simulink model "population_fractal"  (Simulink 7.1)
settings: Solver=ode45  StartTime=0.0  StopTime=600.0  RelTol=1e-3
libraries: simulink x1
settings Model: Creator=Usuario  LastModifiedBy=Usuario

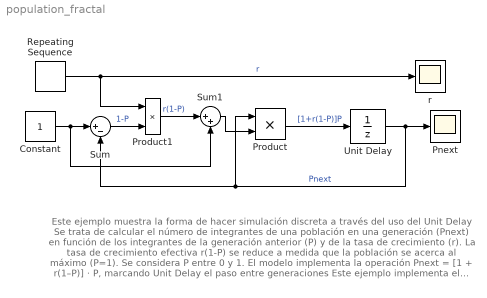
== system population_fractal ==
  note: Este ejemplo muestra la forma de hacer simulación discreta a través del uso del Unit Delay
      | Se trata de calcular el número de integrantes de una población en una generación (Pnext) en función de los integrantes
      | de la generación anterior (P) y de la tasa de crecimiento (r). La tasa de crecimiento efectiva r(1-P) se reduce a medida que la
      | población se acerca al máximo (P=1). Se considera P entre 0 y 1.
      | El modelo implementa la operación Pnext = [1 + r(1–P)] · P, marcando Unit Delay el paso entre generaciones
      |
      | Este ejemplo implementa el Fractal de Feigenbaum, conocido ejemplo introductorio a la Teoría del Caos y la Bifurcación
      | http://library.thinkquest.org/26242/full/ap/ap16.html
  Constant : Constant  OutDataType=sfix(16)  OutScaling=2^0
  Pnext : Scope
  Product : Product  OutDataType=sfix(16)  OutScaling=2^0  RndMeth=Zero
  Product1 : Product  OutDataType=sfix(16)  OutScaling=2^0  RndMeth=Zero
  Repeating Sequence : simulink/Sources/Repeating Sequence  SystemSampleTime=-1  rep_seq_t=[0 100 101 200 201 300 301 400 401 500 501 600]  rep_seq_y=[1.75 1.75 2 2 2.25 2.25 2.5 2.5 2.75 2.75 3 3]
  Sum : Sum  Inputs=|+-  OutDataType=sfix(16)  OutScaling=2^0
  Sum1 : Sum  Inputs=|++  OutDataType=sfix(16)  OutScaling=2^0
  Unit Delay : UnitDelay  X0=0.5
  r : Scope
  wires:
  Unit Delay/1 -> Pnext/1, Sum/2, Product/1  "Pnext"
  Constant/1 -> Sum/1, Sum1/2
  Sum/1 -> Product1/2  "1-P"
  Product1/1 -> Sum1/1  "r(1-P)"
  Sum1/1 -> Product/2
  Product/1 -> Unit Delay/1  "[1+r(1-P)]P"
  Repeating Sequence/1 -> Product1/1, r/1  "r"
